simulink model "simulator"  (R2023b)
settings: configuration reference "SharedConfiguration" (kept outside this file)
undefined symbols (not defined in the file or in its folder): DiscIntNeverNeededParam
libraries: simulink x20
(part 2 of 2)

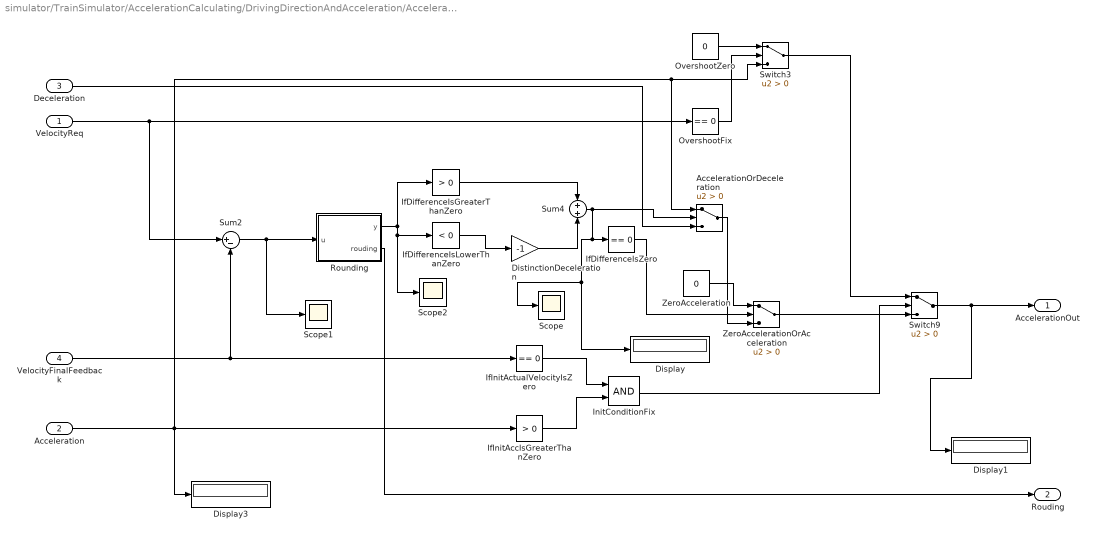
== system simulator/TrainSimulator/AccelerationCalculating/DrivingDirectionAndAcceleration/Acceleration ==
  VelocityReq : Inport  OutDataTypeStr=double
  Acceleration : Inport  Port=2  OutDataTypeStr=double
  Deceleration : Inport  Port=3  OutDataTypeStr=double
  VelocityFinalFeedback : Inport  Port=4  OutDataTypeStr=double
  AccelerationOrDeceleration : Switch  Criteria=u2 > Threshold  OutDataTypeStr=double  SaturateOnIntegerOverflow=off  InputSameDT=off
  Display : Display
  Display1 : Display
  Display3 : Display
  DistinctionDeceleration : Gain  Gain=-1  ParamDataTypeStr=double  OutDataTypeStr=int8
  IfDifferenceIsGreaterThanZero : simulink/Logic and Bit Operations/Compare To Zero  relop=>  OutDataTypeStr=boolean
      settings: LibrarySourceBlock=|
      | simulink/Quick Insert/Logic and Bit
      | Operations/IsZero
  IfDifferenceIsLowerThanZero : simulink/Logic and Bit Operations/Compare To Zero  relop=<  OutDataTypeStr=boolean
      settings: LibrarySourceBlock=|
      | simulink/Quick Insert/Logic and Bit
      | Operations/IsZero
  IfDifferenceIsZero : simulink/Logic and Bit Operations/Compare To Zero  relop===  OutDataTypeStr=boolean
      settings: LibrarySourceBlock=|
      | simulink/Quick Insert/Logic and Bit
      | Operations/IsZero
  IfInitAccIsGreaterThanZero : simulink/Logic and Bit Operations/Compare To Zero  relop=>  OutDataTypeStr=boolean
      settings: LibrarySourceBlock=|
      | simulink/Quick Insert/Logic and Bit
      | Operations/IsZero
  IfInitActualVelocityIsZero : simulink/Logic and Bit Operations/Compare To Zero  relop===  OutDataTypeStr=boolean
      settings: LibrarySourceBlock=|
      | simulink/Quick Insert/Logic and Bit
      | Operations/IsZero
  InitConditionFix : Logic  AllPortsSameDT=off  OutDataTypeStr=boolean
  OvershootFix : simulink/Logic and Bit Operations/Compare To Zero  relop===  OutDataTypeStr=boolean
      settings: LibrarySourceBlock=|
      | simulink/Quick Insert/Logic and Bit
      | Operations/IsZero
  OvershootZero : Constant  Value=0  OutDataTypeStr=int8
  Rounding : MATLAB Function  TreatAsAtomicUnit=on
  Scope : Scope
  Scope1 : Scope
  Scope2 : Scope
  Sum2 : Sum  Inputs=|+-  OutDataTypeStr=double  AccumDataTypeStr=double
  Sum4 : Sum  OutDataTypeStr=double  AccumDataTypeStr=int8  RndMeth=Round
  Switch3 : Switch  Criteria=u2 > Threshold  OutDataTypeStr=double  SaturateOnIntegerOverflow=off  InputSameDT=off
  Switch9 : Switch  Criteria=u2 > Threshold  OutDataTypeStr=double  SaturateOnIntegerOverflow=off  InputSameDT=off
  ZeroAcceleration : Constant  Value=0  OutDataTypeStr=uint8
  ZeroAccelerationOrAcceleration : Switch  Criteria=u2 > Threshold  OutDataTypeStr=double  SaturateOnIntegerOverflow=off  InputSameDT=off
  AccelerationOut : Outport  OutDataTypeStr=double  OutputWhenDisabled=reset  InitialOutput=0
  Rouding : Outport  Port=2  OutDataTypeStr=double
  wires:
  AccelerationOrDeceleration/1 -> ZeroAccelerationOrAcceleration/3
  ZeroAccelerationOrAcceleration/1 -> Switch9/3
  Acceleration/1 -> Display3/1, AccelerationOrDeceleration/1, Switch3/3, IfInitAccIsGreaterThanZero/1
  Rounding/1(y) -> Scope2/1, IfDifferenceIsLowerThanZero/1, IfDifferenceIsGreaterThanZero/1
  IfInitAccIsGreaterThanZero/1 -> InitConditionFix/2
  Sum2/1 -> Scope1/1, Rounding/1(u)
  VelocityFinalFeedback/1 -> IfInitActualVelocityIsZero/1, Sum2/2
  ZeroAcceleration/1 -> ZeroAccelerationOrAcceleration/1
  IfDifferenceIsLowerThanZero/1 -> DistinctionDeceleration/1
  VelocityReq/1 -> Sum2/1, OvershootFix/1
  IfDifferenceIsGreaterThanZero/1 -> Sum4/1
  Sum4/1 -> AccelerationOrDeceleration/2, IfDifferenceIsZero/1, Scope/1, Display/1
  DistinctionDeceleration/1 -> Sum4/2
  InitConditionFix/1 -> Switch9/2
  Switch9/1 -> Display1/1, AccelerationOut/1
  Deceleration/1 -> AccelerationOrDeceleration/3
  IfInitActualVelocityIsZero/1 -> InitConditionFix/1
  Switch3/1 -> Switch9/1
  OvershootFix/1 -> Switch3/2
  OvershootZero/1 -> Switch3/1
  IfDifferenceIsZero/1 -> ZeroAccelerationOrAcceleration/2
  Rounding/2(rouding) -> Rouding/1

== system simulator/TrainSimulator/AccelerationCalculating/DrivingDirectionAndAcceleration/Deceleration ==
  VelocityFinalFeedback : Inport  OutDataTypeStr=double
  DecelerationIn : Inport  Port=2  OutDataTypeStr=double
  IfSpeedIsZero : simulink/Logic and Bit Operations/Compare To Constant  relop===  const=0  OutDataTypeStr=boolean
  IsSpeedGreaterThanZero : simulink/Logic and Bit Operations/Compare To Zero  relop=>  OutDataTypeStr=boolean
      settings: LibrarySourceBlock=|
      | simulink/Quick Insert/Logic and Bit
      | Operations/IsZero
  OneForEnable : Constant  OutDataTypeStr=uint8
  Scope : Scope
  Switch5 : Switch  Criteria=u2 > Threshold  OutDataTypeStr=double  SaturateOnIntegerOverflow=off  InputSameDT=off
  SwitchForReset : Switch  Criteria=u2 > Threshold  OutDataTypeStr=uint8  SaturateOnIntegerOverflow=off  InputSameDT=off
  ZeroDeceleration : Constant  Value=0  OutDataTypeStr=uint8
  ZeroForEnable : Constant  Value=0  OutDataTypeStr=uint8
  DecelerationOut : Outport  OutDataTypeStr=double
  ResetSelectionOfDirection : Outport  Port=2  OutDataTypeStr=uint8
  wires:
  Switch5/1 -> IfSpeedIsZero/1, DecelerationOut/1
  DecelerationIn/1 -> Switch5/1
  IsSpeedGreaterThanZero/1 -> Switch5/2
  ZeroDeceleration/1 -> Switch5/3
  VelocityFinalFeedback/1 -> Scope/1, IsSpeedGreaterThanZero/1
  IfSpeedIsZero/1 -> SwitchForReset/2
  ZeroForEnable/1 -> SwitchForReset/1
  OneForEnable/1 -> SwitchForReset/3
  SwitchForReset/1 -> ResetSelectionOfDirection/1

== system simulator/TrainSimulator/AccelerationCalculating/DrivingDirectionAndAcceleration/SelectNominalOrReverseDirectionAndHold ==
  DirectionIn : Inport  OutDataTypeStr=uint8
  ChangeDirectionIn : Inport  Port=2  OutDataTypeStr=uint8
  ChangeDirection : Subsystem  TreatAsAtomicUnit=on
  Delay One Step : Delay  DelayLength=1  InitialConditionSource=Input port
      settings: InputPortMap=u0,p4
  IfDirectionIsSet : simulink/Logic and Bit Operations/Compare To Constant  relop===  const=0  OutDataTypeStr=boolean
  Scope : Scope
  SwitchAndHold : Switch  Criteria=u2 > Threshold  OutDataTypeStr=uint8  SaturateOnIntegerOverflow=off  InputSameDT=off
  DirectionOut : Outport  OutDataTypeStr=uint8
  wires:
  SwitchAndHold/1 -> DirectionOut/1, Delay One Step/1
  Delay One Step/1 -> IfDirectionIsSet/1, SwitchAndHold/3
  ChangeDirection/1(ChDout) -> SwitchAndHold/2
  IfDirectionIsSet/1 -> Scope/1, ChangeDirection/1(ChDIn)
  DirectionIn/1 -> Delay One Step/2, SwitchAndHold/1
  ChangeDirectionIn/1 -> ChangeDirection/Enable

== system simulator/TrainSimulator/AccelerationCalculating/DrivingDirectionAndAcceleration/SelectNominalOrReverseDirectionAndHold/ChangeDirection ==
  ChDIn : Inport  OutDataTypeStr=boolean
  Enable : EnablePort
  ChDout : Outport  OutDataTypeStr=boolean  OutputWhenDisabled=reset  InitialOutput=1
  wires:
  ChDIn/1 -> ChDout/1

== matlab function simulator/TrainSimulator/AccelerationCalculating/DrivingDirectionAndAcceleration/Acceleration/Rounding ==
  data: u input; y output; rouding output
function [y, rouding] = fcn(u)

y = u;
if (y > - 0.005) && (y < 0.005)
    y = 0;
    rouding = 1;
else 
    rouding = 0;
end
end

== matlab function simulator/TrainSimulator/AccToForceAndForceToAcc/TractionCharacteristics/ZeroReplacedByDecimal ==
  data: u input; y output
function y = fcn(u)

y = u;
if (y == 0)
    y = 0.000000001;
end
end

== matlab function simulator/TrainSimulator/AccToForceAndForceToAcc/TractionCharacteristics/LimitMaxAcceleration ==
  data: u1 input; y1 output; u2 input; y2 output
function [y1,y2] = fcn(u1,u2)

y1 = u1;
y2 = u2;

if (y1 > 2)
    y1 = 2;
end

if (y2 > 2)
    y2 = 2;
end
end

== matlab function simulator/TrainSimulator/ConfidenceInterval/ConfidenceIntervalCalculation ==
  data: DistanceIn input; DistanceOut output; CI_Overreading input; CI_Underreading input; CI_OverreadingOut output; CI_UnderreadingOut output; CI_AfterReset input; Reset input; nSamples data_store_memory; CI_Over data_store_memory; CI_Under data_store_memory; DistanceLastSample data_store_memory
function [DistanceOut,CI_OverreadingOut,CI_UnderreadingOut]  = fcn(DistanceIn,CI_Overreading,CI_Underreading,CI_AfterReset,Reset)

global DistanceLastSample;
global nSamples;
global CI_Over;
global CI_Under;
double distance_growth;

if Reset == 1 
    nSamples = 0;
end

nSamples = nSamples + 1;

if nSamples == 1
    CI_Init = CI_AfterReset * DistanceIn; 
    CI_Over =  CI_Init;
    CI_Under = CI_Init;
else
    distance_growth = abs(DistanceIn - DistanceLastSample);
    CI_Over = CI_Over + (CI_Overreading * distance_growth);
    CI_Under = CI_Under + (CI_Underreading * distance_growth); 
end

DistanceLastSample = DistanceIn;
DistanceOut = DistanceIn;
CI_OverreadingOut = DistanceIn - CI_Over;
CI_UnderreadingOut = DistanceIn + CI_Under;
end
